simulink model "washing_machine_test1"  (R2024b)
settings: Solver=VariableStepAuto  StartTime=0.0  StopTime=inf  RelTol=1e-3
settings Model: Creator=sunil  LastModifiedBy=sunil

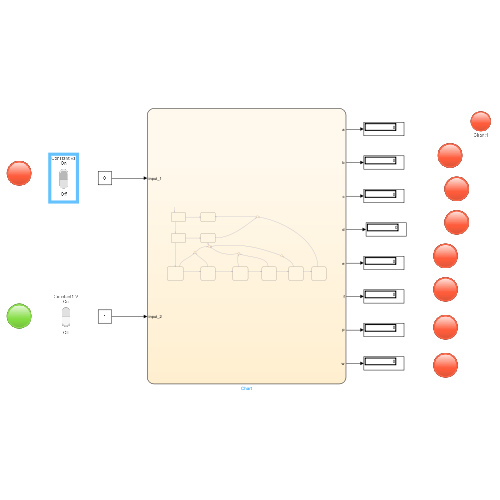
[thumbnail: Simulink's stored preview of the top-level diagram]
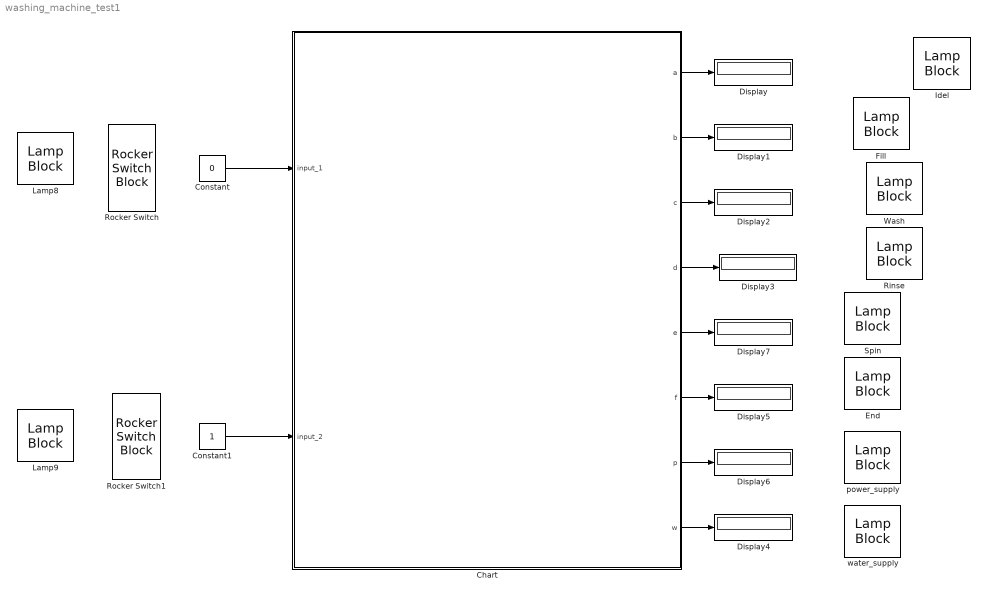
== system washing_machine_test1 ==
  Chart : Stateflow chart  TreatAsAtomicUnit=on
  Constant : Constant  Value=0
  Constant1 : Constant
  Display{,1..7} (8 alike) : Display
  End : LampBlock  LabelPosition=Hide
  Fill : LampBlock  LabelPosition=Hide
  Idel : LampBlock  LabelPosition=Bottom
  Lamp8 : LampBlock  LabelPosition=Hide
  Lamp9 : LampBlock  LabelPosition=Hide
  Rinse : LampBlock  LabelPosition=Hide
  Rocker Switch : RockerSwitchBlock
      settings: Values={{'Off', 'On'}, [0 1]}
  Rocker Switch1 : RockerSwitchBlock
      settings: Values={{'Off', 'On'}, [0 1]}
  Spin : LampBlock  LabelPosition=Hide
  Wash : LampBlock  LabelPosition=Hide
  power_supply : LampBlock  LabelPosition=Hide
  water_supply : LampBlock  LabelPosition=Hide
  wires:
  Constant/1 -> Chart/1(input_1)
  Constant1/1 -> Chart/2(input_2)
  Chart/1(a) -> Display/1
  Chart/2(b) -> Display1/1
  Chart/3(c) -> Display2/1
  Chart/4(d) -> Display3/1
  Chart/8(w) -> Display4/1
  Chart/6(f) -> Display5/1
  Chart/7(p) -> Display6/1
  Chart/5(e) -> Display7/1

== stateflow chart washing_machine_test1/Chart ==
  state power_on
    entry:
    p=1;
  state power_off
    entry:
    p=0;
    f=0;
  state water_on
    entry:
    w=1;
  state water_off
    entry:
    w=0
  state end
    entry:
    f=1;
    exit:
    p=0
  state ideal
    entry:
    a=1
    exit:
    a=0;
  state fill
    entry:
    b=1;
    exit:
    b=0;
  state wash
    entry:
    c=1;
    exit:
    c=0;
    w=0;
  state Rinse
    entry:
    d=1
    exit:
    d=0
  state spin
    entry:
    e=1;
    exit:
    e=0
  (default) -> power_on
  (junction 20) -> power_off
  power_on -> power_off [order 2]
  end -> (junction 20)
  water_off -> (junction 20)
  power_on -> water_on [order 1] : [input_1==1]
  water_on -> water_off [order 2]
  water_on -> ideal [order 1] : [input_2==1]
  (junction 35) -> water_off
  (junction 31) -> (junction 35)
  (junction 27) -> (junction 35)
  (junction 30) -> (junction 35)
  ideal -> (junction 27) [order 2] : [input_1==0||input_2==0]
  fill -> (junction 27) [order 2] : [input_1==0||input_2==0]
  Rinse -> (junction 30) [order 2] : [input_1==0||input_2==0]
  wash -> (junction 30) [order 2] : [input_1==0||input_2==0]
  spin -> (junction 31) [order 2] : [input_1==0||input_2==0]
  spin -> end [order 1] : [after(5,sec)]
  ideal -> fill [order 1] : [after(5,sec)]
  fill -> wash [order 1] : [after(5,sec)]
  wash -> Rinse [order 1] : [after(5,sec)]
  Rinse -> spin [order 1] : [after(5,sec)]
  data: a output; b output; c output; d output; e output; f output; p output; w output; input_1 input; input_2 input
